simulink model "MotorTorqueControlTest_working_5_8_2022_ADC_FILT_Mo"  (R2024b)
settings: Solver=FixedStepAuto  StartTime=0.0  StopTime=inf  FixedStep=0.001  RelTol=1e-3  EnableMultiTasking=on
undefined symbols (not defined in the file): mu_X, mu_y, sigma_X, sigma_y
libraries: slrealtimeethercatlib x35, slrealtimeiplib x6, slrealtimeutilitieslib x5, simulink_extras x5, slrealtimeloglib x3, slpidlib x1, simulink x1
(part 2 of 4)

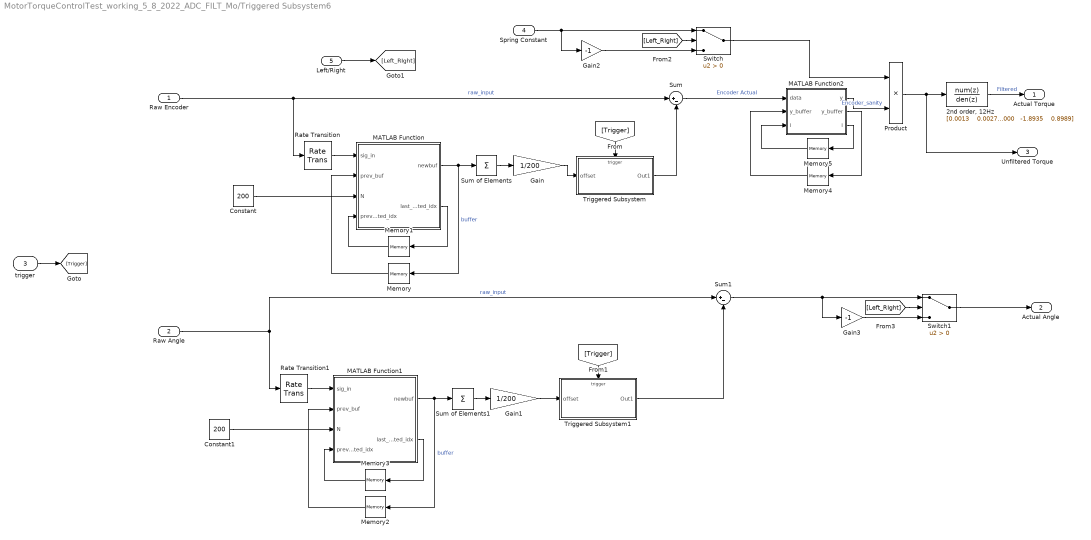
== system MotorTorqueControlTest_working_5_8_2022_ADC_FILT_Mo/Triggered Subsystem6 ==
  Raw Encoder : Inport
  Raw Angle : Inport  Port=2
  trigger : Inport  Port=3
  Spring Constant : Inport  Port=4
  Left/Right : Inport  Port=5
  "2nd order, 12Hz" : DiscreteFilter  Numerator="[0.0013    0.0027    0.0013]"  Denominator="[1.0000   -1.8935    0.8989]"
  Constant : Constant  Value=200
  Constant1 : Constant  Value=200
  Gain : Gain  Gain=1/200
  Gain1 : Gain  Gain=1/200
  Gain2 : Gain  Gain=-1
  Gain3 : Gain  Gain=-1
  MATLAB Function : MATLAB Function  TreatAsAtomicUnit=on  SystemSampleTime=1/200
  MATLAB Function1 : MATLAB Function  TreatAsAtomicUnit=on  SystemSampleTime=1/200
  MATLAB Function2 : MATLAB Function  TreatAsAtomicUnit=on
  Memory : Memory  InitialCondition=zeros(200,1)
  Memory1 : Memory
  Memory2 : Memory  InitialCondition=zeros(200,1)
  Memory3 : Memory
  Memory4 : Memory  InitialCondition=zeros(1,5)
  Memory5 : Memory
  Product : Product
  Rate Transition : RateTransition  OutPortSampleTime=1/200
  Rate Transition1 : RateTransition  OutPortSampleTime=1/200
  Sum : Sum  Inputs=|+-
  Sum of Elements : Sum  Inputs=+
  Sum of Elements1 : Sum  Inputs=+
  Sum1 : Sum  Inputs=|+-
  Switch : Switch  Criteria=u2 > Threshold  SaturateOnIntegerOverflow=off  InputSameDT=off
  Switch1 : Switch  Criteria=u2 > Threshold  SaturateOnIntegerOverflow=off  InputSameDT=off
  Triggered Subsystem : Subsystem  TreatAsAtomicUnit=on
  Triggered Subsystem1 : Subsystem  TreatAsAtomicUnit=on
  Actual Torque : Outport
  Actual Angle : Outport  Port=2
  Unfiltered Torque : Outport  Port=3
  wires:
  Rate Transition/1 -> MATLAB Function/1(sig_in)
  Memory1/1 -> MATLAB Function/4(prev_updated_idx)
  MATLAB Function/2(last_updated_idx) -> Memory1/1
  Memory/1 -> MATLAB Function/2(prev_buf)
  Constant/1 -> MATLAB Function/3(N)
  Sum of Elements/1 -> Gain/1
  Triggered Subsystem/1(Out1) -> Sum/2
  Gain/1 -> Triggered Subsystem/1(offset)
  MATLAB Function/1(newbuf) -> Memory/1, Sum of Elements/1  "buffer"
  Raw Encoder/1 -> Sum/1, Rate Transition/1  "raw_input"
  MATLAB Function1/2(last_updated_idx) -> Memory3/1
  [Trigger] -> Triggered Subsystem1/Trigger
  Memory2/1 -> MATLAB Function1/2(prev_buf)
  Gain1/1 -> Triggered Subsystem1/1(offset)
  Sum of Elements1/1 -> Gain1/1
  MATLAB Function1/1(newbuf) -> Memory2/1, Sum of Elements1/1  "buffer"
  Constant1/1 -> MATLAB Function1/3(N)
  Rate Transition1/1 -> MATLAB Function1/1(sig_in)
  Raw Angle/1 -> Sum1/1, Rate Transition1/1  "raw_input"
  Memory3/1 -> MATLAB Function1/4(prev_updated_idx)
  trigger/1 -> [Trigger]
  [Trigger] -> Triggered Subsystem/Trigger
  Triggered Subsystem1/1(Out1) -> Sum1/2
  Sum1/1 -> Gain3/1, Switch1/1
  Sum/1 -> MATLAB Function2/1(data)  "Encoder Actual"
  Product/1 -> Unfiltered Torque/1, "2nd order, 12Hz"/1
  Spring Constant/1 -> Gain2/1, Switch/1
  Memory4/1 -> MATLAB Function2/2("y_buffer ")
  "2nd order, 12Hz"/1 -> Actual Torque/1  "Filtered"
  Left/Right/1 -> [Left_RIght]
  Gain2/1 -> Switch/3
  Switch/1 -> Product/1
  Gain3/1 -> Switch1/3
  Switch1/1 -> Actual Angle/1
  [Left_RIght] -> Switch/2
  [Left_RIght] -> Switch1/2
  MATLAB Function2/2(y_buffer) -> Memory4/1
  MATLAB Function2/1(y) -> Product/2  "Encoder_sanity"
  MATLAB Function2/3(i) -> Memory5/1
  Memory5/1 -> MATLAB Function2/3("i ")

== system MotorTorqueControlTest_working_5_8_2022_ADC_FILT_Mo/RL-AAN/Triggered Subsystem ==
  note: Note: Add input/output of Critic Loss, Actor Loss, Uc, Eta, V_tderr
  In1 : Inport
  Trigger : TriggerPort  VariantControl=(inherit)
  Byte Packing : slrealtimeutilitieslib/Byte Packing  MaskPackedDataType=uint8  MaskUnpackedDataTypes={'double'}  MaskAlignment=1
  UDP Send : slrealtimeiplib/UDP Send  useHostTargetConn=off  toAddress='192.168.7.15'  toPort=5555  sampleTime=-1  enableMessage=off
  bytes : Constant  Value=8
  wires:
  Byte Packing/1 -> UDP Send/1
  bytes/1 -> UDP Send/2
  In1/1 -> Byte Packing/1

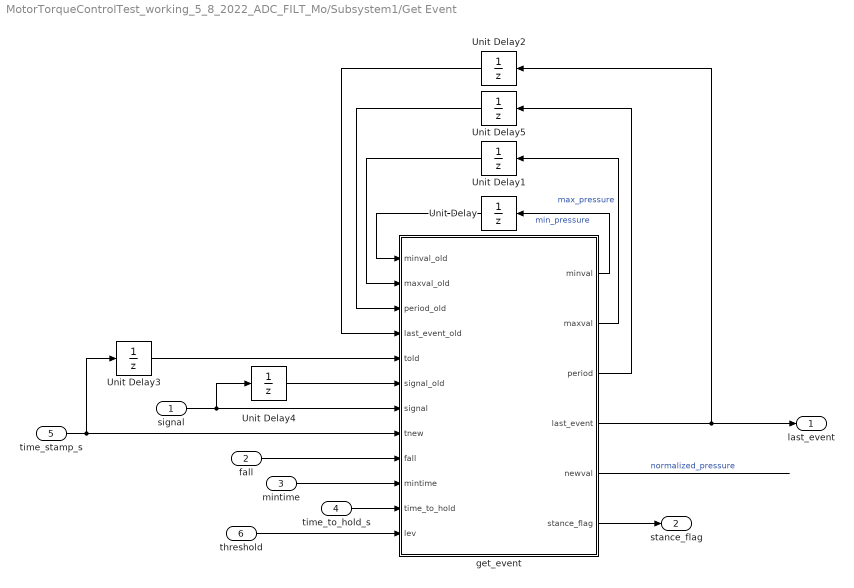
== system MotorTorqueControlTest_working_5_8_2022_ADC_FILT_Mo/Subsystem1/Get Event ==
  signal : Inport
  fall : Inport  Port=2
  mintime : Inport  Port=3
  time_to_hold_s : Inport  Port=4
  time_stamp_s : Inport  Port=5
  threshold : Inport  Port=6
  Unit Delay : UnitDelay  InitialCondition=50  SampleTime=-1
  Unit Delay1 : UnitDelay  InitialCondition=400  SampleTime=-1
  Unit Delay{2..5} (4 alike) : UnitDelay  SampleTime=-1
  get_event : MATLAB Function  TreatAsAtomicUnit=on
  last_event : Outport
  stance_flag : Outport  Port=2
  wires:
  get_event/6(stance_flag) -> stance_flag/1
  get_event/5(newval) -> ?  "normalized_pressure"
  time_stamp_s/1 -> Unit Delay3/1, get_event/8(tnew)
  Unit Delay5/1 -> get_event/3(period_old)
  signal/1 -> Unit Delay4/1, get_event/7(signal)
  get_event/3(period) -> Unit Delay5/1
  threshold/1 -> get_event/12(lev)
  Unit Delay4/1 -> get_event/6(signal_old)
  Unit Delay3/1 -> get_event/5(told)
  fall/1 -> get_event/9(fall)
  mintime/1 -> get_event/10(mintime)
  time_to_hold_s/1 -> get_event/11(time_to_hold)
  Unit Delay2/1 -> get_event/4(last_event_old)
  Unit Delay1/1 -> get_event/2(maxval_old)
  Unit Delay/1 -> get_event/1(minval_old)
  get_event/4(last_event) -> Unit Delay2/1, last_event/1
  get_event/2(maxval) -> Unit Delay1/1  "max_pressure"
  get_event/1(minval) -> Unit Delay/1  "min_pressure"

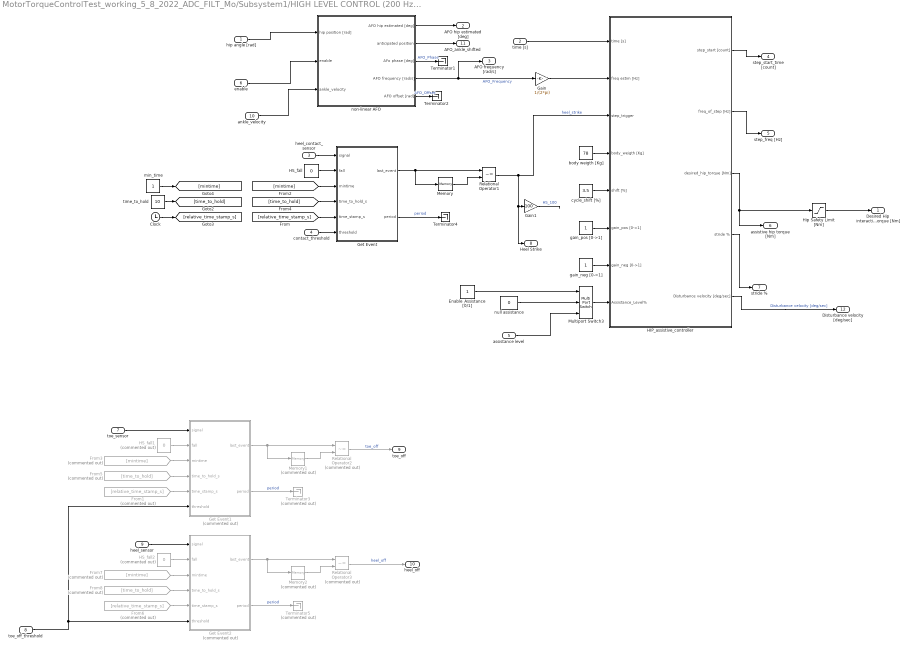
== system MotorTorqueControlTest_working_5_8_2022_ADC_FILT_Mo/Subsystem1/HIGH LEVEL CONTROL (200 Hz)1 ==
  hip angle [rad] : Inport
  time [s] : Inport  Port=2
  heel_contact_sensor : Inport  Port=3
  contact_threshold : Inport  Port=4
  assistance level : Inport  Port=5
  enable : Inport  Port=6
  toe_sensor : Inport  Port=7
  toe_off_threshold : Inport  Port=8
  heel_sensor : Inport  Port=9
  ankle_velocity : Inport  Port=10
  Clock : Clock
  Enable_Assistance [0/1] : Constant  OutMin=[0]  OutMax=[1]  SampleTime=0.01
  From1 : From  Commented=on  GotoTag=relative_time_stamp_s
      settings: CloseFcn=tagdialog Close
  From3 : From  Commented=on  GotoTag=mintime
      settings: CloseFcn=tagdialog Close
  From5 : From  Commented=on  GotoTag=time_to_hold
      settings: CloseFcn=tagdialog Close
  From6 : From  Commented=on  GotoTag=relative_time_stamp_s
      settings: CloseFcn=tagdialog Close
  From7 : From  Commented=on  GotoTag=mintime
      settings: CloseFcn=tagdialog Close
  From8 : From  Commented=on  GotoTag=time_to_hold
      settings: CloseFcn=tagdialog Close
  Gain : Gain  Gain=1/(2*pi)
  Gain1 : Gain  Gain=100
  Get Event : Subsystem  TreatAsAtomicUnit=on  SystemSampleTime=1/200
  Get Event1 : Subsystem  Commented=on  TreatAsAtomicUnit=on  SystemSampleTime=1/200
  Get Event2 : Subsystem  Commented=on  TreatAsAtomicUnit=on  SystemSampleTime=1/200
  HIP_assistive_controller : Subsystem
  HS_fall : Constant  Value=0
  HS_fall1 : Constant  Commented=on  Value=0
  HS_fall2 : Constant  Commented=on  Value=0
  Hip Safety Limit [Nm] : Saturate  UpperLimit=50  LowerLimit=-50  SampleTime=0.01
  Memory : Memory
  Memory1 : Memory  Commented=on
  Memory2 : Memory  Commented=on
  Multiport Switch3 : MultiPortSwitch  DataPortOrder=Zero-based contiguous  Inputs=2  zeroidx=on  SampleTime=0.01  SaturateOnIntegerOverflow=off  InputSameDT=off
  Relational Operator1 : RelationalOperator  Operator=~=  OutDataTypeStr=boolean  RndMeth=Simplest  InputSameDT=off
  Relational Operator2 : RelationalOperator  Commented=on  Operator=~=  OutDataTypeStr=boolean  RndMeth=Simplest  InputSameDT=off
  Relational Operator3 : RelationalOperator  Commented=on  Operator=~=  OutDataTypeStr=boolean  RndMeth=Simplest  InputSameDT=off
  Terminator1 : Terminator
  Terminator2 : Terminator
  Terminator3 : Terminator  Commented=on
  Terminator4 : Terminator
  Terminator5 : Terminator  Commented=on
  body weigth [Kg] : Constant  Value=78  OutMin=[0]  OutMax=[100]  SampleTime=0.01
  cycle_shift [%] : Constant  Value=3.5  SampleTime=0.01
  gain_neg [0->1] : Constant  OutMin=[0]  OutMax=[1]  SampleTime=0.01
  gain_pos [0->1] : Constant  OutMin=[0]  OutMax=[1]  SampleTime=0.01
  min_time : Constant
  non-linear AFO : Subsystem
  null assistance : Constant  Value=0  OutMin=[0]  OutMax=[1]  SampleTime=0.01
  time_to_hold : Constant  Value=10
  Desired Hip interaction Torque [Nm] : Outport
  AFO hip estimated [deg] : Outport  Port=2
  AFO frequency [rad/s] : Outport  Port=3
  step_start_time [count] : Outport  Port=4
  step_freq [Hz] : Outport  Port=5
  assistive hip torque [Nm] : Outport  Port=6
  stride % : Outport  Port=7
  Heel Strike : Outport  Port=8
  toe_off : Outport  Port=9
  heel_off : Outport  Port=10
  AFO_ankle_shifted : Outport  Port=11
  Disturbance velocity [deg/sec] : Outport  Port=12
  wires:
  HIP_assistive_controller/5(Disturbance velocity [deg/sec]) -> Disturbance velocity [deg/sec]/1  "Disturbance velocity [deg/sec]"
  ankle_velocity/1 -> non-linear AFO/3(ankle_velocity)
  Get Event2/2(period) -> Terminator5/1  "period"
  From8/1 -> Get Event2/4(time_to_hold_s)
  Memory2/1 -> Relational Operator3/2
  Relational Operator3/1 -> heel_off/1  "heel_off"
  heel_sensor/1 -> Get Event2/1(signal)
  Get Event2/1(last_event) -> Relational Operator3/1, Memory2/1
  From7/1 -> Get Event2/3(mintime)
  From6/1 -> Get Event2/5(time_stamp_s)
  toe_off_threshold/1 -> Get Event1/6(threshold), Get Event2/6(threshold)
  HS_fall2/1 -> Get Event2/2(fall)
  Relational Operator2/1 -> toe_off/1  "toe_off"
  From5/1 -> Get Event1/4(time_to_hold_s)
  Memory1/1 -> Relational Operator2/2
  Get Event1/1(last_event) -> Relational Operator2/1, Memory1/1
  HS_fall1/1 -> Get Event1/2(fall)
  From1/1 -> Get Event1/5(time_stamp_s)
  toe_sensor/1 -> Get Event1/1(signal)
  Get Event1/2(period) -> Terminator3/1  "period"
  From3/1 -> Get Event1/3(mintime)
  enable/1 -> non-linear AFO/2(enable)
  Gain1/1 -> ?  "HS_100"
  hip angle [rad]/1 -> non-linear AFO/1(hip position [rad])
  heel_contact_sensor/1 -> Get Event/1(signal)
  time_to_hold/1 -> [time_to_hold]
  [relative_time_stamp_s] -> Get Event/5(time_stamp_s)
  [mintime] -> Get Event/3(mintime)
  [time_to_hold] -> Get Event/4(time_to_hold_s)
  contact_threshold/1 -> Get Event/6(threshold)
  Clock/1 -> [relative_time_stamp_s]
  min_time/1 -> [mintime]
  Get Event/2(period) -> Terminator4/1  "period"
  Get Event/1(last_event) -> Relational Operator1/1, Memory/1
  Memory/1 -> Relational Operator1/2
  Relational Operator1/1 -> HIP_assistive_controller/3(step_trigger), Gain1/1, Heel Strike/1  "heel_strike"
  HS_fall/1 -> Get Event/2(fall)
  assistance level/1 -> Multiport Switch3/3
  Multiport Switch3/1 -> HIP_assistive_controller/8(Assistance_Level%)
  gain_pos [0->1]/1 -> HIP_assistive_controller/6(gain_pos [0->1])
  non-linear AFO/5(AFO offset [rad]) -> Terminator2/1  "AFO_Offset"
  non-linear AFO/3(AFo phase [deg]) -> Terminator1/1  "AFO_Phase"
  non-linear AFO/2(anticipated position) -> AFO_ankle_shifted/1
  null assistance/1 -> Multiport Switch3/2
  Enable_Assistance [0/1]/1 -> Multiport Switch3/1
  gain_neg [0->1]/1 -> HIP_assistive_controller/7(gain_neg [0->1])
  cycle_shift [%]/1 -> HIP_assistive_controller/5(shift [%])
  body weigth [Kg]/1 -> HIP_assistive_controller/4(body_weigth [Kg])
  HIP_assistive_controller/4(stride %) -> stride %/1
  HIP_assistive_controller/3(desired_hip_torque [Nm]) -> assistive hip torque [Nm]/1, Hip Safety Limit [Nm]/1
  HIP_assistive_controller/2(freq_of_step [Hz]) -> step_freq [Hz]/1
  HIP_assistive_controller/1(step_start [count]) -> step_start_time [count]/1
  time [s]/1 -> HIP_assistive_controller/1(time [s])
  Gain/1 -> HIP_assistive_controller/2(freq estim [Hz])
  non-linear AFO/4(AFO frequency [rad/s]) -> AFO frequency [rad/s]/1, Gain/1  "AFO_Frequency"
  non-linear AFO/1(AFO hip estimated [deg]) -> AFO hip estimated [deg]/1
  Hip Safety Limit [Nm]/1 -> Desired Hip interaction Torque [Nm]/1

== system MotorTorqueControlTest_working_5_8_2022_ADC_FILT_Mo/Subsystem1/stride % calculation ==
  step_trigger : Inport
  timer : Inport  Port=2
  step_freq_estimated : Inport  Port=3
  Product1 : Product  RndMeth=Zero
  Sum : Sum  Inputs=|-+
  take step start and period : Subsystem  TreatAsAtomicUnit=on
  to% : Gain  Gain=100
  stride % : Outport
  wires:
  to%/1 -> stride %/1
  step_trigger/1 -> take step start and period/Trigger
  timer/1 -> take step start and period/1(time_counter), Sum/2
  take step start and period/1(time_count_stepon) -> Sum/1
  step_freq_estimated/1 -> Product1/2
  Sum/1 -> Product1/1
  Product1/1 -> to%/1

== system MotorTorqueControlTest_working_5_8_2022_ADC_FILT_Mo/Triggered Subsystem6/Triggered Subsystem ==
  offset : Inport
  Trigger : TriggerPort  VariantControl=(inherit)
  Out1 : Outport
  wires:
  offset/1 -> Out1/1

== system MotorTorqueControlTest_working_5_8_2022_ADC_FILT_Mo/Triggered Subsystem6/Triggered Subsystem1 ==
  offset : Inport
  Trigger : TriggerPort  VariantControl=(inherit)
  Out1 : Outport
  wires:
  offset/1 -> Out1/1

== system MotorTorqueControlTest_working_5_8_2022_ADC_FILT_Mo/Subsystem1/HIGH LEVEL CONTROL (200 Hz)1/Get Event ==
  signal : Inport
  fall : Inport  Port=2
  mintime : Inport  Port=3
  time_to_hold_s : Inport  Port=4
  time_stamp_s : Inport  Port=5
  threshold : Inport  Port=6
  Unit Delay{,2..5} (5 alike) : UnitDelay  SampleTime=-1
  Unit Delay1 : UnitDelay  InitialCondition=-1000  SampleTime=-1
  get_event : MATLAB Function  TreatAsAtomicUnit=on
  last_event : Outport
  period : Outport  Port=2
  wires:
  get_event/5(newval) -> ?  "normalized_pressure"
  time_stamp_s/1 -> Unit Delay3/1, get_event/8(tnew)
  Unit Delay5/1 -> get_event/3(period_old)
  signal/1 -> Unit Delay4/1, get_event/7(signal)
  get_event/3(period) -> Unit Delay5/1, period/1
  threshold/1 -> get_event/12(lev)
  Unit Delay4/1 -> get_event/6(signal_old)
  Unit Delay3/1 -> get_event/5(told)
  fall/1 -> get_event/9(fall)
  mintime/1 -> get_event/10(mintime)
  time_to_hold_s/1 -> get_event/11(time_to_hold)
  Unit Delay2/1 -> get_event/4(last_event_old)
  Unit Delay1/1 -> get_event/2(maxval_old)
  Unit Delay/1 -> get_event/1(minval_old)
  get_event/4(last_event) -> Unit Delay2/1, last_event/1
  get_event/2(maxval) -> Unit Delay1/1  "max_pressure"
  get_event/1(minval) -> Unit Delay/1  "min_pressure"

== system MotorTorqueControlTest_working_5_8_2022_ADC_FILT_Mo/Subsystem1/HIGH LEVEL CONTROL (200 Hz)1/Get Event1 ==
  signal : Inport
  fall : Inport  Port=2
  mintime : Inport  Port=3
  time_to_hold_s : Inport  Port=4
  time_stamp_s : Inport  Port=5
  threshold : Inport  Port=6
  Unit Delay : UnitDelay  InitialCondition=4.5  SampleTime=-1
  Unit Delay1 : UnitDelay  InitialCondition=0.5  SampleTime=-1
  Unit Delay{2..5} (4 alike) : UnitDelay  SampleTime=-1
  get_event : MATLAB Function  TreatAsAtomicUnit=on
  last_event : Outport
  period : Outport  Port=2
  wires:
  time_stamp_s/1 -> Unit Delay3/1, get_event/8(tnew)
  Unit Delay5/1 -> get_event/3(period_old)
  signal/1 -> Unit Delay4/1, get_event/7(signal)
  get_event/3(period) -> period/1, Unit Delay5/1
  threshold/1 -> get_event/12(lev)
  Unit Delay4/1 -> get_event/6(signal_old)
  Unit Delay3/1 -> get_event/5(told)
  fall/1 -> get_event/9(fall)
  mintime/1 -> get_event/10(mintime)
  time_to_hold_s/1 -> get_event/11(time_to_hold)
  Unit Delay2/1 -> get_event/4(last_event_old)
  Unit Delay1/1 -> get_event/2(maxval_old)
  Unit Delay/1 -> get_event/1(minval_old)
  get_event/4(last_event) -> last_event/1, Unit Delay2/1
  get_event/2(maxval) -> Unit Delay1/1
  get_event/1(minval) -> Unit Delay/1

== system MotorTorqueControlTest_working_5_8_2022_ADC_FILT_Mo/Subsystem1/HIGH LEVEL CONTROL (200 Hz)1/Get Event2 ==
  signal : Inport
  fall : Inport  Port=2
  mintime : Inport  Port=3
  time_to_hold_s : Inport  Port=4
  time_stamp_s : Inport  Port=5
  threshold : Inport  Port=6
  Unit Delay : UnitDelay  InitialCondition=4.5  SampleTime=-1
  Unit Delay1 : UnitDelay  InitialCondition=0.5  SampleTime=-1
  Unit Delay{2..5} (4 alike) : UnitDelay  SampleTime=-1
  get_event : MATLAB Function  TreatAsAtomicUnit=on
  last_event : Outport
  period : Outport  Port=2
  wires:
  time_stamp_s/1 -> Unit Delay3/1, get_event/8(tnew)
  Unit Delay5/1 -> get_event/3(period_old)
  signal/1 -> Unit Delay4/1, get_event/7(signal)
  get_event/3(period) -> period/1, Unit Delay5/1
  threshold/1 -> get_event/12(lev)
  Unit Delay4/1 -> get_event/6(signal_old)
  Unit Delay3/1 -> get_event/5(told)
  fall/1 -> get_event/9(fall)
  mintime/1 -> get_event/10(mintime)
  time_to_hold_s/1 -> get_event/11(time_to_hold)
  Unit Delay2/1 -> get_event/4(last_event_old)
  Unit Delay1/1 -> get_event/2(maxval_old)
  Unit Delay/1 -> get_event/1(minval_old)
  get_event/4(last_event) -> last_event/1, Unit Delay2/1
  get_event/2(maxval) -> Unit Delay1/1
  get_event/1(minval) -> Unit Delay/1

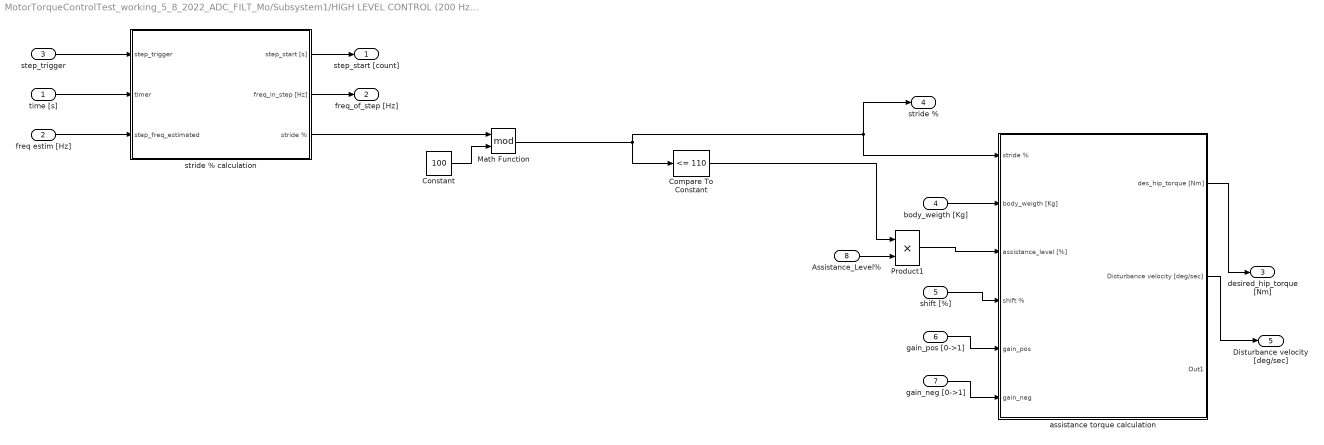
== system MotorTorqueControlTest_working_5_8_2022_ADC_FILT_Mo/Subsystem1/HIGH LEVEL CONTROL (200 Hz)1/HIP_assistive_controller ==
  time [s] : Inport
  freq estim [Hz] : Inport  Port=2
  step_trigger : Inport  Port=3
  body_weigth [Kg] : Inport  Port=4
  shift [%] : Inport  Port=5
  gain_pos [0->1] : Inport  Port=6
  gain_neg [0->1] : Inport  Port=7
  Assistance_Level% : Inport  Port=8
  Compare To Constant : simulink/Logic and Bit Operations/Compare To Constant  relop=<=  const=110  OutDataTypeStr=uint8
  Constant : Constant  Value=100
  Math Function : Math  Operator=mod
  Product1 : Product  RndMeth=Zero  SampleTime=0.01
  assistance torque calculation : Subsystem
  stride % calculation : Subsystem
  step_start [count] : Outport
  freq_of_step [Hz] : Outport  Port=2
  desired_hip_torque [Nm] : Outport  Port=3
  stride % : Outport  Port=4
  Disturbance velocity [deg/sec] : Outport  Port=5
  wires:
  assistance torque calculation/2(Disturbance velocity [deg/sec]) -> Disturbance velocity [deg/sec]/1
  Constant/1 -> Math Function/2
  stride % calculation/3(stride %) -> Math Function/1
  Assistance_Level%/1 -> Product1/2
  Product1/1 -> assistance torque calculation/3(assistance_level [%])
  gain_neg [0->1]/1 -> assistance torque calculation/6(gain_neg)
  gain_pos [0->1]/1 -> assistance torque calculation/5(gain_pos)
  shift [%]/1 -> assistance torque calculation/4(shift %)
  Compare To Constant/1 -> Product1/1
  assistance torque calculation/1(des_hip_torque [Nm]) -> desired_hip_torque [Nm]/1
  freq estim [Hz]/1 -> stride % calculation/3(step_freq_estimated)
  stride % calculation/2(freq_in_step [Hz]) -> freq_of_step [Hz]/1
  time [s]/1 -> stride % calculation/2(timer)
  stride % calculation/1(step_start [s]) -> step_start [count]/1
  step_trigger/1 -> stride % calculation/1(step_trigger)
  Math Function/1 -> Compare To Constant/1, stride %/1, assistance torque calculation/1(stride %)
  body_weigth [Kg]/1 -> assistance torque calculation/2(body_weigth [Kg])

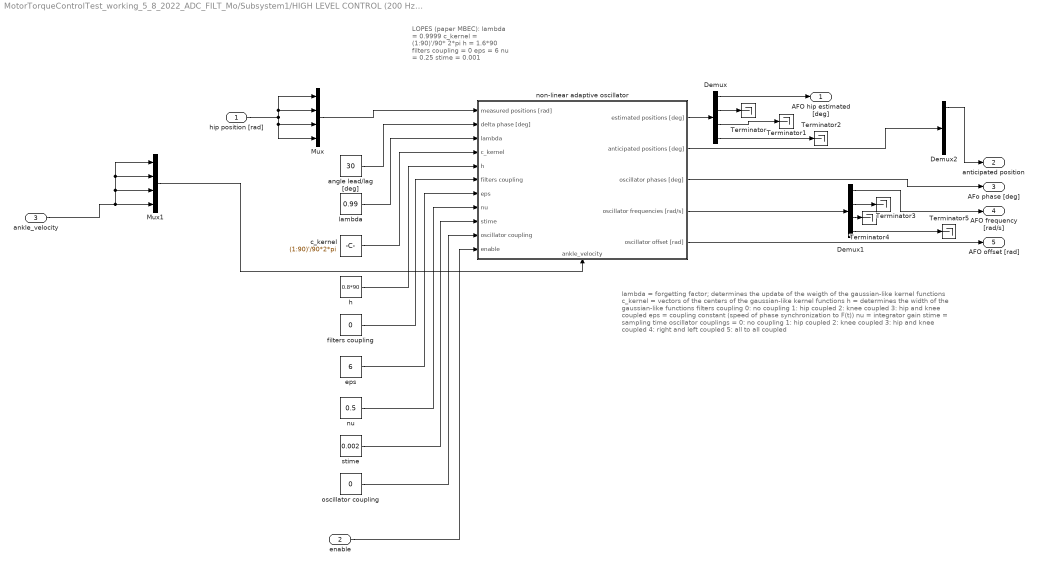
== system MotorTorqueControlTest_working_5_8_2022_ADC_FILT_Mo/Subsystem1/HIGH LEVEL CONTROL (200 Hz)1/non-linear AFO ==
  note: lambda = forgetting factor; determines the update of the weigth of the gaussian-like kernel functions
      | c_kernel = vectors of the centers of the gaussian-like kernel functions
      | h = determines the width of the gaussian-like functions
      | filters coupling
      | 0: no coupling
      | 1: hip coupled
      | 2: knee coupled
      | 3: hip and knee coupled
      | eps = coupling constant (speed of phase synchronization to F(t))
      | nu = integrator gain
      | stime = sampling time
      | oscillator couplings =
      | 0: no coupling
      | 1: hip coupled
      | 2: knee coupled
      | 3: hip and knee coupled
      | 4: right and left coupled
      | 5: all to all coupled
  note: LOPES (paper MBEC):
      | lambda = 0.9999
      | c_kernel = (1:90)'/90* 2*pi
      | h = 1.6*90
      | filters coupling = 0
      | eps = 6
      | nu = 0.25
      | stime = 0.001
  hip position [rad] : Inport
  enable : Inport  Port=2
  ankle_velocity : Inport  Port=3
  Demux : Demux
  Demux1 : Demux
  Demux2 : Demux
  Mux : Mux
  Mux1 : Mux
  Terminator{,1..5} (6 alike) : Terminator
  angle lead/lag [deg] : Constant  Value=30  SampleTime=0.01
  c_kernel : Constant  Value=(1:90)'/90*2*pi  SampleTime=0.01
  eps : Constant  Value=6  SampleTime=0.01
  filters coupling : Constant  Value=0  SampleTime=0.01
  h : Constant  Value=0.8*90  SampleTime=0.01
  lambda : Constant  Value=0.99  SampleTime=0.01
  non-linear adaptive oscillator : Subsystem
      settings: PortSchema="{\"entries\":[{\"content\":{\"sides\":[{\"content\":{\"connectorIds\":[\"In1\",\"In2\",\"In3\",\"In4\",\"In5\",\"In6\",\"In7\",\"In8\",\"In9\",\"In10\",\"In11\"]},\"type\":\"ConnectorPlacement.EquallySpacedRectSide\",\"uuid\":\"ab3a5fe0-9bb0-482e-b44f-9f3ccb1731cf\"},{\"content\":{\"connectorIds\":[\"Out1\",\"Out2\",\"Out3\",\"Out4\",\"Out5\"],\"side\":\"RIGHT\"},\"type\":\"ConnectorPlacement.EquallySpacedRectSide\",\"uuid\":\"96980b87-f654-464e-8cdf-49c302ee1131\"},{\"content\":{\"connectorIds\":[],\"side\":\"TOP\"},\"type\":\"ConnectorPlacement.EquallySpacedRectSide\",\"uuid\":\"71bd0918-5e69-4492-a5e8-d47966924c89\"},{\"content\":{\"connectorIds\":[\"In12\"],\"side\":\"BOTTOM\"},\"type\":\"ConnectorPlacement.EquallySpacedRectSide\",\"uuid\":\"e65d897a-cb77-4120-a9be-e238fcdd4933\"}]},\"type\":\"ConnectorPlacement.EquallySpacedConnector\",\"uuid\":\"727f1d0f-0b0c-4f59-bcfa-1816f6ded572\"}],\"packageUris\":[\"http://schema.mathworks.com/mf0/Connector/R2020b\"],\"version\":\"1.0\"}"
  nu : Constant  Value=0.5  SampleTime=0.01
  oscillator coupling : Constant  Value=0  SampleTime=0.01
  stime : Constant  Value=0.002  SampleTime=0.01
  AFO hip estimated [deg] : Outport
  anticipated position : Outport  Port=2
  AFo phase [deg] : Outport  Port=3
  AFO frequency [rad/s] : Outport  Port=4
  AFO offset [rad] : Outport  Port=5
  wires:
  Mux1/1 -> non-linear adaptive oscillator/12(ankle_velocity)
  ankle_velocity/1 -> Mux1/4, Mux1/2, Mux1/1, Mux1/3
  Demux2/1 -> anticipated position/1
  enable/1 -> non-linear adaptive oscillator/11(enable)
  Demux1/4 -> Terminator5/1
  Demux1/3 -> Terminator4/1
  Demux1/2 -> Terminator3/1
  Demux/4 -> Terminator2/1
  Demux/3 -> Terminator1/1
  Demux/2 -> Terminator/1
  Demux1/1 -> AFO frequency [rad/s]/1
  non-linear adaptive oscillator/4(oscillator frequencies [rad/s]) -> Demux1/1
  non-linear adaptive oscillator/5(oscillator offset [rad]) -> AFO offset [rad]/1
  non-linear adaptive oscillator/3(oscillator phases [deg]) -> AFo phase [deg]/1
  non-linear adaptive oscillator/2(anticipated positions [deg]) -> Demux2/1
  hip position [rad]/1 -> Mux/3, Mux/4, Mux/2, Mux/1
  Demux/1 -> AFO hip estimated [deg]/1
  non-linear adaptive oscillator/1(estimated positions [deg]) -> Demux/1
  Mux/1 -> non-linear adaptive oscillator/1(measured positions [rad])
  oscillator coupling/1 -> non-linear adaptive oscillator/10(oscillator coupling)
  nu/1 -> non-linear adaptive oscillator/8(nu)
  stime/1 -> non-linear adaptive oscillator/9(stime)
  eps/1 -> non-linear adaptive oscillator/7(eps)
  filters coupling/1 -> non-linear adaptive oscillator/6(filters coupling)
  h/1 -> non-linear adaptive oscillator/5(h)
  c_kernel/1 -> non-linear adaptive oscillator/4(c_kernel)
  lambda/1 -> non-linear adaptive oscillator/3(lambda)
  angle lead/lag [deg]/1 -> non-linear adaptive oscillator/2(delta phase [deg])

== system MotorTorqueControlTest_working_5_8_2022_ADC_FILT_Mo/Subsystem1/stride % calculation/take step start and period ==
  time_counter : Inport
  Trigger : TriggerPort  VariantControl=(inherit)
  time_count_stepon : Outport
  wires:
  time_counter/1 -> time_count_stepon/1

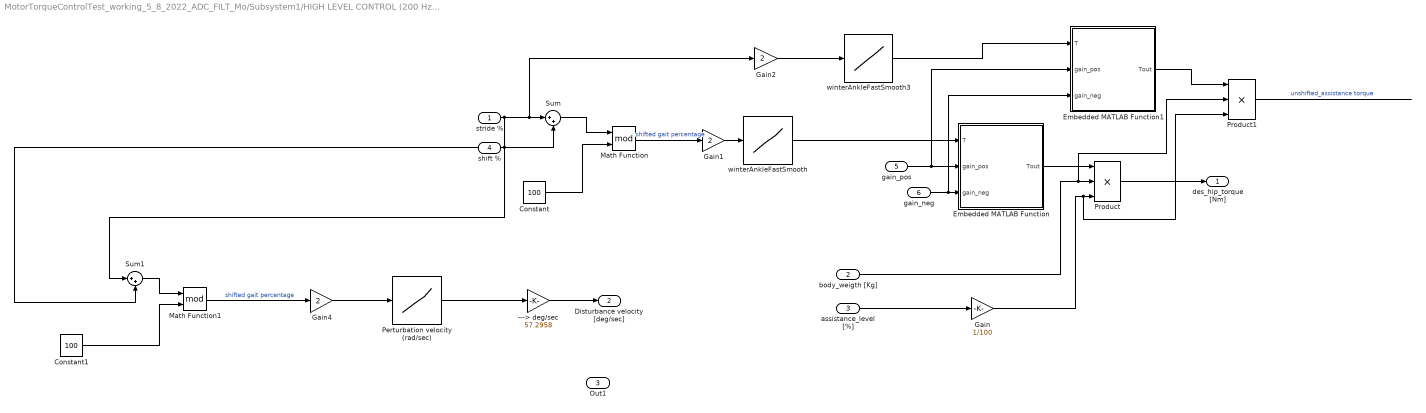
== system MotorTorqueControlTest_working_5_8_2022_ADC_FILT_Mo/Subsystem1/HIGH LEVEL CONTROL (200 Hz)1/HIP_assistive_controller/assistance torque calculation ==
  stride % : Inport
  body_weigth [Kg] : Inport  Port=2
  assistance_level [%] : Inport  Port=3
  shift % : Inport  Port=4
  gain_pos : Inport  Port=5
  gain_neg : Inport  Port=6
  ---> deg/sec : Gain  Gain=57.2958
  Constant : Constant  Value=100
  Constant1 : Constant  Value=100
  Embedded MATLAB Function : MATLAB Function  TreatAsAtomicUnit=on
  Embedded MATLAB Function1 : MATLAB Function  TreatAsAtomicUnit=on
  Gain : Gain  Gain=1/100  SampleTime=0.01
  Gain1 : Gain  Gain=2
  Gain2 : Gain  Gain=2
  Gain4 : Gain  Gain=2
  Math Function : Math  Operator=mod
  Math Function1 : Math  Operator=mod
  Perturbation velocity (rad/sec) : Lookup  InputValues=[0:199]  Table="[-4.93270593173997e-253\t4.04481886402677e-252\t-2.92815289519947e-249\t2.11997865130555e-246\t-1.53486161539233e-243\t1.11123768956540e-240\t-8.04534552383726e-238\t5.82481904688132e-235\t-4.21716094459655e-232\t3.05321869906885e-229\t-2.21052612096491e-226\t1.60041785835989e-223\t-1.15870031892643e-220\t8.38897430484885e-218\t-6.07360580970738e-215\t4.39728221725384e-212\t-3.18362625168597e-209\t2.30494100893842e-206\t-1.66877410684517e-203\t1.20819014841489e-200\t-8.74727998678275e-198\t6.33301862852906e-195\t-4.58509673977517e-192\t3.31960370657860e-189\t-2.40338849846610e-186\t1.74004995328580e-183\t-1.25979376279042e-180\t9.12088944210309e-178\t-6.60351135814501e-175\t4.78093310240728e-172\t-3.46138896263170e-169\t2.50604082801225e-166\t-1.81437009809191e-163\t1.31360144497771e-160\t-9.51045631793764e-158\t6.88555723817240e-155\t-4.98513392998050e-152\t3.60923007974864e-149\t-2.61307759260409e-146\t1.89186456781528e-143\t-1.36970733402067e-140\t9.91666217966397e-138\t-7.17964972100335e-135\t5.19805648134426e-132\t-3.76338571284352e-129\t2.72468605804223e-126\t-1.97266894263686e-123\t1.42820958978303e-120\t-1.03402177033392e-117\t7.48630333512205e-115\t-5.42007327441066e-112\t3.92412556436998e-109\t-2.84106148853059e-106\t2.05692459357058e-103\t-1.48921056468361e-100\t1.07818639190634e-97\t-7.80605458529627e-95\t5.65157273789058e-92\t-4.09173085617816e-89\t2.96240748830027e-86\t-2.14477892979854e-83\t1.55281698276666e-80\t-1.12423735074413e-77\t8.13946289121766e-75\t-5.89295989086808e-72\t4.26649482152560e-69\t-3.08893635782464e-66\t2.23638565657022e-63\t-1.61914012642048e-60\t1.17225521514277e-57\t-8.48711156623239e-55\t6.14465705140010e-52\t-4.44872321810211e-49\t3.22086946524887e-46\t-2.33190504411696e-43\t1.68829603107122e-40\t-1.22232399459052e-37\t8.84960883787503e-35\t-6.40710457538158e-32\t4.63873486296742e-29\t-3.35843763368384e-26\t2.43150420805224e-23\t-1.76040568819219e-20\t1.27453128674693e-17\t-9.22758891199092e-15\t6.68076162696856e-12\t-4.83686219033632e-09\t3.50188154504187e-06\t-0.00626761298606990\t-0.0765669636741737\t-0.159007648472814\t-0.255697732492699\t-0.366569255690371\t-0.490682383459649\t-0.627060602245939\t-0.775477718863351\t-0.936729568178100\t-1.11230265194788\t-1.30336585588083\t-1.50962253596126\t-1.72869176641761\t-1.95637366717679\t-2.18811628055900\t-2.42034717099672\t-2.65047734470819\t-2.87635971143045\t-3.09600015053043\t-3.30729754329227\t-3.50752844204451\t-3.69318852845936\t-3.86078591589950\t-4.00765115546246\t-4.13182288263306\t-4.23158106680777\t-4.30521091005464\t-4.35074237213917\t-4.36540997346769\t-4.34542368201912\t-4.28664128375527\t-4.18519646810363\t-4.03727504299778\t-3.83904583007861\t-3.58777079098347\t-3.28337600797458\t-2.93062745352010\t-1.28036789819353\t0.00132410560966730\t-1.82887864053534e-06\t2.52608028950714e-09\t-3.48906782965580e-12\t4.81916365465694e-15\t-6.65631608906347e-18\t9.19382429245723e-21\t-1.26986765636748e-23\t1.75396419747845e-26\t-2.42260710445788e-29\t3.34614879311990e-32\t-4.62176129389610e-35\t6.38366037447886e-38\t-8.81722728314056e-41\t1.21785139562475e-43\t-1.68211839640513e-46\t2.32337238327194e-49\t-3.20908399960916e-52\t4.43244491958885e-55\t-6.12217317078076e-58\t8.45605642325827e-61\t-1.16796582257095e-63\t1.61321553974235e-66\t-2.22820251018784e-69\t3.07763364788833e-72\t-4.25088331393000e-75\t5.87139699393623e-78\t-8.10967982758677e-81\t1.12012366007425e-83\t-1.54713507873650e-86\t2.13693098108324e-89\t-2.95156775945036e-92\t4.07675882644125e-95\t-5.63089309935420e-98\t7.77749149415344e-101\t-1.07424120604507e-103\t1.48376140254605e-106\t-2.04939811217073e-109\t2.83066577615762e-112\t-3.90976681822861e-115\t5.40024071428065e-118\t-7.45891024400900e-121\t1.03023818699522e-123\t-1.42298363597511e-126\t1.96545076062331e-129\t-2.71471617436249e-132\t3.74961512900386e-135\t-5.17903630163337e-138\t7.15337870443307e-141\t-9.88037617594962e-144\t1.36469544549312e-146\t-1.88494205664256e-149\t2.60351609484272e-152\t-3.59602356593311e-155\t4.96689285399923e-158\t-6.86036233377885e-161\t9.47565665984445e-164\t-1.30879485319833e-166\t1.80773114650458e-169\t-2.49687098788397e-172\t3.44872341342956e-175\t-4.76343921654497e-178\t6.57934848626995e-181\t-9.08751524600982e-184\t1.25518405840322e-186\t-1.73368294612913e-189\t2.39459427290897e-192\t-3.30745696302266e-195\t4.56831943766322e-198\t-6.30984551510508e-201\t8.71527286298032e-204\t-1.20376926652754e-206\t1.66266790505841e-209\t-2.29673474975219e-212]"  SaturateOnIntegerOverflow=off
  Product : Product  Inputs=3  RndMeth=Zero
  Product1 : Product  Inputs=3  RndMeth=Zero
  Sum : Sum  Inputs=|++
  Sum1 : Sum  Inputs=|++
  winterAnkleFastSmooth : Lookup  InputValues=[0:200]  Table="[0\t0\t0\t0\t0\t0\t0\t0\t0\t0\t0\t0\t0\t0\t0\t0\t0\t0\t0.0123629052736435\t0.0412585090601981\t0.0720000000000000\t0.104333911147289\t0.137883548612989\t0.172241411772194\t0.207000000000000\t0.241722256560577\t0.275852900274400\t0.308807093851024\t0.340000000000000\t0.368933312610405\t0.395454850289409\t0.419498962823709\t0.441000000000000\t0.459966367997805\t0.476702698567963\t0.491587679854139\t0.505000000000000\t0.517248090398375\t0.528359355438741\t0.538290942759736\t0.547000000000000\t0.554463145408695\t0.560734879677075\t0.565889174106917\t0.570000000000000\t0.573149327966846\t0.575451125852960\t0.577027360812594\t0.578000000000000\t0.578502042723923\t0.578710616911085\t0.578813882642705\t0.579000000000000\t0.579451876137464\t0.580331406502699\t0.581795233616584\t0.584000000000000\t0.587112327726223\t0.591338757078120\t0.596895807890957\t0.604000000000000\t0.612880062957646\t0.623813565184823\t0.637090284819588\t0.653000000000000\t0.671711170443192\t0.692906982182590\t0.716149302830693\t0.741000000000000\t0.767228380269585\t0.795433506084817\t0.826421878857641\t0.861000000000000\t0.899672183478468\t0.941733993478140\t0.986178806738742\t1.03200000000000\t1.07844226081654\t1.12575552000262\t1.17444101918739\t1.22500000000000\t1.27765252325536\t1.33149392651137\t1.38533836651170\t1.43800000000000\t1.48843202116203\t1.53614377395190\t1.58078363976582\t1.62200000000000\t1.65933814209653\t1.69193097768103\t1.71880832442502\t1.73900000000000\t1.75165291045186\t1.75638231532399\t1.75292056253412\t1.74100000000000\t1.72026896609601\t1.69003976102303\t1.64954067543852\t1.59800000000000\t1.53500560016408\t1.46158364058391\t1.37911986071179\t1.28900000000000\t1.19256800824768\t1.09100067664133\t0.985433006714323\t0.877000000000000\t0.767175491845209\t0.658788652850752\t0.555007487430919\t0.459000000000000\t0.373308149371486\t0.297969711955659\t0.232396418562003\t0.176000000000000\t0.128170035668849\t0.0882074993266129\t0.0553912133210702\t0.0290000000000000\t0.00830858295311821\t-0.00742470926211037\t-0.0189456468462838\t-0.0270000000000000\t-0.0322793674813219\t-0.0352586622781714\t-0.0363586259359352\t-0.0360000000000000\t-0.0345973630278306\t-0.0325406416252041\t-0.0302135994099755\t-0.0280000000000000\t-0.0261905554073556\t-0.0247037712210123\t-0.0233651014241628\t-0.0220000000000000\t-0.0204841653427468\t-0.0188942734907467\t-0.0173572448933732\t-0.0160000000000000\t-0.0149196582216572\t-0.0140941348160010\t-0.0134715440023443\t-0.0130000000000000\t-0.0126340767706245\t-0.0123541872452493\t-0.0121472040972494\t-0.0120000000000000\t-0.0119034096958447\t-0.0118641162030018\t-0.0118927646086579\t-0.0120000000000000\t-0.0121897844459966\t-0.0124393479427436\t-0.0127192374681188\t-0.0130000000000000\t-0.0132593275201690\t-0.0135034920260239\t-0.0137459105188668\t-0.0140000000000000\t-0.0142729054733275\t-0.0145466839531609\t-0.0147971204564139\t-0.0150000000000000\t-0.0151334255865212\t-0.0151847721613325\t-0.0151437326554777\t-0.0150000000000000\t-0.0147402671805879\t-0.0143392274015089\t-0.0137685739216755\t-0.0130000000000000\t-0.0120148806911273\t-0.0108333182326318\t-0.00948509665782044\t-0.00800000000000000\t-0.00640333505490292\t-0.00470249966796380\t-0.00290041444704278\t-0.00100000000000000\t0.000987595910738992\t0.00301831690448703\t0.00503987944599156\t0.00700000000000000\t0.00884357641194696\t0.0105042320500157\t0.0119127716630766\t0.0130000000000000\t0.0137162234414732\t0.0140897548954503\t0.0141684089017022\t0.0140000000000000\t0.0136196548221603\t0.0130117483681832\t0.0121479677301145\t0.0110000000000000\t0.00953953226988547\t0.00773825163181676\t0.00556784517783966\t0.00300000000000000]"  SaturateOnIntegerOverflow=off
  winterAnkleFastSmooth3 : Lookup  InputValues=[0:200]  Table=|  SaturateOnIntegerOverflow=off
      | [-0.00700000000000000
      | -0.00198044104598932
      | -0.00904907548113065
      | -0.0250931721757067
      | -0.0470000000000000
      | -0.0716568278242934
      | -0.0959509245188694
      | -0.116769558954011
      | -0.131000000000000
      | -0.136360997656837
      | -0.133897226443392
      | -0.125484842008251
      | -0.113000000000000
      | -0.0979929315483575
      | -0.0807101697075629
      | -0.0610723230129869
      | -0.0390000000000000
      | -0.0144641511497329
      | 0.0123629052736435
      | 0.0412585090601981
      | 0.0720000000000000
      | 0.104333911147289
      | 0.137883548612989
      | 0.172241411772194
      | 0.207000000000000
      | 0.241722256560577
      | 0.275852900274400
      | 0.308807093851024
      | 0.340000000000000
      | 0.368933312610405
      | 0.395454850289409
      | 0.419498962823709
      | 0.441000000000000
      | 0.459966367997805
      | 0.476702698567963
      | 0.491587679854139
      | 0.505000000000000
      | 0.517248090398375
      | 0.528359355438741
      | 0.538290942759736
      | 0.547000000000000
      | 0.554463145408695
      | 0.560734879677075
      | 0.565889174106917
      | 0.570000000000000
      | 0.573149327966846
      | 0.575451125852960
      | 0.577027360812594
      | 0.578000000000000
      | 0.578502042723923
      | 0.578710616911085
      | 0.578813882642705
      | 0.579000000000000
      | 0.579451876137464
      | 0.580331406502699
      | 0.581795233616584
      | 0.584000000000000
      | 0.587112327726223
      | 0.591338757078120
      | 0.596895807890957
      | 0.604000000000000
      | 0.612880062957646
      | 0.623813565184823
      | 0.637090284819588
      | 0.653000000000000
      | 0.671711170443192
      | 0.692906982182590
      | 0.716149302830693
      | 0.741000000000000
      | 0.767228380269585
      | 0.795433506084817
      | 0.826421878857641
      | 0.861000000000000
      | 0.899672183478468
      | 0.941733993478140
      | 0.986178806738742
      | 1.03200000000000
      | 1.07844226081654
      | 1.12575552000262
      | 1.17444101918739
      | 1.22500000000000
      | 1.27765252325536
      | 1.33149392651137
      | 1.38533836651170
      | 1.43800000000000
      | 1.48843202116203
      | 1.53614377395190
      | 1.58078363976582
      | 1.62200000000000
      | 1.65933814209653
      | 1.69193097768103
      | 1.71880832442502
      | 1.73900000000000
      | 1.75165291045186
      | 1.75638231532399
      | 1.75292056253412
      | 1.74100000000000
      | 1.72026896609601
      | 1.69003976102303
      | 1.64954067543852
      | 1.59800000000000
      | 1.53500560016408
      | 1.46158364058391
      | 1.37911986071179
      | 1.28900000000000
      | 1.19256800824768
      | 1.09100067664133
      | 0.985433006714323
      | 0.877000000000000
      | 0.767175491845209
      | 0.658788652850752
      | 0.555007487430919
      | 0.459000000000000
      | 0.373308149371486
      | 0.297969711955659
      | 0.232396418562003
      | 0.176000000000000
      | 0.128170035668849
      | 0.0882074993266129
      | 0.0553912133210702
      | 0.0290000000000000
      | 0.00830858295311821
      | -0.00742470926211037
      | -0.0189456468462838
      | -0.0270000000000000
      | -0.0322793674813219
      | -0.0352586622781714
      | -0.0363586259359352
      | -0.0360000000000000
      | -0.0345973630278306
      | -0.0325406416252041
      | -0.0302135994099755
      | -0.0280000000000000
      | -0.0261905554073556
      | -0.0247037712210123
      | -0.0233651014241628
      | -0.0220000000000000
      | -0.0204841653427468
      | -0.0188942734907467
      | -0.0173572448933732
      | -0.0160000000000000
      | -0.0149196582216572
      | -0.0140941348160010
      | -0.0134715440023443
      | -0.0130000000000000
      | -0.0126340767706245
      | -0.0123541872452493
      | -0.0121472040972494
      | -0.0120000000000000
      | -0.0119034096958447
      | -0.0118641162030018
      | -0.0118927646086579
      | -0.0120000000000000
      | -0.0121897844459966
      | -0.0124393479427436
      | -0.0127192374681188
      | -0.0130000000000000
      | -0.0132593275201690
      | -0.0135034920260239
      | -0.0137459105188668
      | -0.0140000000000000
      | -0.0142729054733275
      | -0.0145466839531609
      | -0.0147971204564139
      | -0.0150000000000000
      | -0.0151334255865212
      | -0.0151847721613325
      | -0.0151437326554777
      | -0.0150000000000000
      | -0.0147402671805879
      | -0.0143392274015089
      | -0.0137685739216755
      | -0.0130000000000000
      | -0.0120148806911273
      | -0.0108333182326318
      | -0.00948509665782044
      | -0.00800000000000000
      | -0.00640333505490292
      | -0.00470249966796380
      | -0.00290041444704278
      | -0.00100000000000000
      | 0.000987595910738992
      | 0.00301831690448703
      | 0.00503987944599156
      | 0.00700000000000000
      | 0.00884357641194696
      | 0.0105042320500157
      | 0.0119127716630766
      | 0.0130000000000000
      | 0.0137162234414732
      | 0.0140897548954503
      | 0.0141684089017022
      | 0.0140000000000000
      | 0.0136196548221603
      | 0.0130117483681832
      | 0.0121479677301145
      | 0.0110000000000000
      | 0.00953953226988547
      | 0.00773825163181676
      | 0.00556784517783966
      | 0.00300000000000000]
  des_hip_torque [Nm] : Outport
  Disturbance velocity [deg/sec] : Outport  Port=2
  Out1 : Outport  Port=3
  wires:
  Sum1/1 -> Math Function1/1
  Math Function1/1 -> Gain4/1  "shifted gait percentage"
  Constant1/1 -> Math Function1/2
  ---> deg/sec/1 -> Disturbance velocity [deg/sec]/1
  Perturbation velocity (rad/sec)/1 -> ---> deg/sec/1
  Gain4/1 -> Perturbation velocity (rad/sec)/1
  Product1/1 -> ?  "unshifted_assistance torque"
  Embedded MATLAB Function1/1(Tout) -> Product1/1
  Gain2/1 -> winterAnkleFastSmooth3/1
  winterAnkleFastSmooth3/1 -> Embedded MATLAB Function1/1(T)
  Math Function/1 -> Gain1/1  "shifted gait percentage"
  Constant/1 -> Math Function/2
  Gain1/1 -> winterAnkleFastSmooth/1
  Product/1 -> des_hip_torque [Nm]/1
  Sum/1 -> Math Function/1
  gain_neg/1 -> Embedded MATLAB Function/3(gain_neg), Embedded MATLAB Function1/3(gain_neg)
  gain_pos/1 -> Embedded MATLAB Function/2(gain_pos), Embedded MATLAB Function1/2(gain_pos)
  Embedded MATLAB Function/1(Tout) -> Product/1
  winterAnkleFastSmooth/1 -> Embedded MATLAB Function/1(T)
  shift %/1 -> Sum1/2, Sum/2
  stride %/1 -> Sum/1, Gain2/1, Sum1/1
  Gain/1 -> Product/3, Product1/3
  assistance_level [%]/1 -> Gain/1
  body_weigth [Kg]/1 -> Product/2, Product1/2

== system MotorTorqueControlTest_working_5_8_2022_ADC_FILT_Mo/Subsystem1/HIGH LEVEL CONTROL (200 Hz)1/HIP_assistive_controller/stride % calculation ==
  step_trigger : Inport
  timer : Inport  Port=2
  step_freq_estimated : Inport  Port=3
  Product1 : Product  RndMeth=Zero
  Sum : Sum  Inputs=|-+
  take step start and period : Subsystem  TreatAsAtomicUnit=on
  to% : Gain  Gain=100  SampleTime=0.01
  step_start [s] : Outport
  freq_in_step [Hz] : Outport  Port=2
  stride % : Outport  Port=3
  wires:
  to%/1 -> stride %/1
  step_trigger/1 -> take step start and period/Trigger
  timer/1 -> take step start and period/1(time_counter), Sum/2
  take step start and period/1(time_count_stepon) -> step_start [s]/1, Sum/1
  step_freq_estimated/1 -> Product1/2, take step start and period/2(actual;_frequency)
  take step start and period/2(frequency for the step) -> freq_in_step [Hz]/1
  Sum/1 -> Product1/1
  Product1/1 -> to%/1

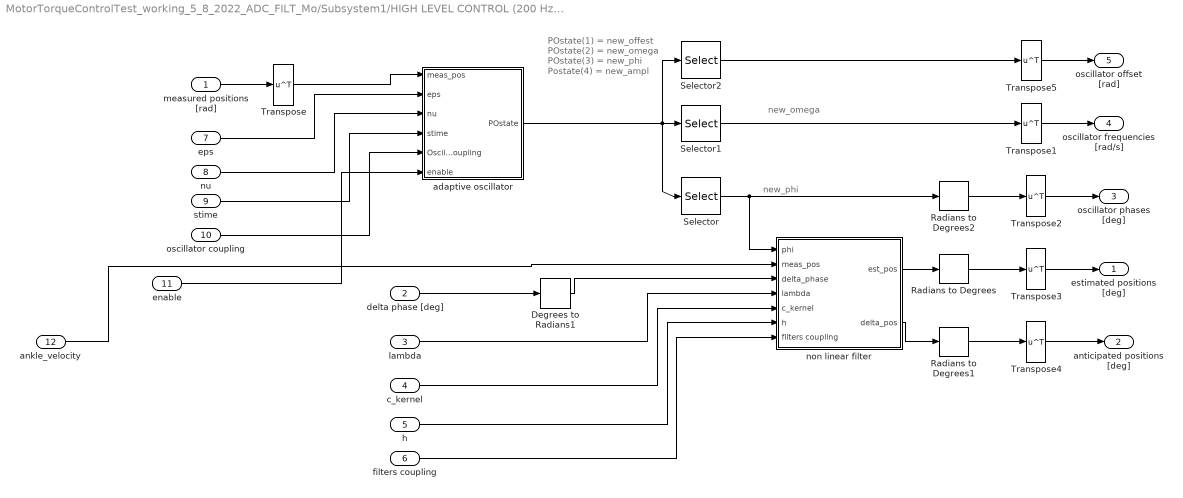
== system MotorTorqueControlTest_working_5_8_2022_ADC_FILT_Mo/Subsystem1/HIGH LEVEL CONTROL (200 Hz)1/non-linear AFO/non-linear adaptive oscillator ==
  note: new_phi
  note: new_omega
  note: POstate(1) = new_offest
      | POstate(2) = new_omega
      | POstate(3) = new_phi
      | Postate(4) = new_ampl
  measured positions [rad] : Inport
  delta phase [deg] : Inport  Port=2
  lambda : Inport  Port=3
  c_kernel : Inport  Port=4
  h : Inport  Port=5
  filters coupling : Inport  Port=6
  eps : Inport  Port=7
  nu : Inport  Port=8
  stime : Inport  Port=9
  oscillator coupling : Inport  Port=10
  enable : Inport  Port=11
  ankle_velocity : Inport  Port=12
  Degrees to Radians1 : simulink_extras/Transformations/Degrees to Radians
  Radians to Degrees : simulink_extras/Transformations/Radians to Degrees
  Radians to Degrees1 : simulink_extras/Transformations/Radians to Degrees
  Radians to Degrees2 : simulink_extras/Transformations/Radians to Degrees
  Selector : Selector  NumberOfDimensions=2  InputPortWidth=3  IndexOptions=Index vector (dialog),Index vector (dialog)  Indices=3,1:4  OutputSizes=1,1
  Selector1 : Selector  NumberOfDimensions=2  InputPortWidth=3  IndexOptions=Index vector (dialog),Index vector (dialog)  Indices=2,1:4  OutputSizes=1,1
  Selector2 : Selector  NumberOfDimensions=2  InputPortWidth=3  IndexOptions=Index vector (dialog),Index vector (dialog)  Indices=1,1:4  OutputSizes=1,1
  Transpose{,1..5} (6 alike) : Math  Operator=transpose
  adaptive oscillator : Subsystem
  non linear filter : Subsystem
  estimated positions [deg] : Outport
  anticipated positions [deg] : Outport  Port=2
  oscillator phases [deg] : Outport  Port=3
  oscillator frequencies [rad/s] : Outport  Port=4
  oscillator offset [rad] : Outport  Port=5
  wires:
  ankle_velocity/1 -> non linear filter/2(meas_pos)
  enable/1 -> adaptive oscillator/6(enable)
  Selector2/1 -> Transpose5/1
  Transpose5/1 -> oscillator offset [rad]/1
  oscillator coupling/1 -> adaptive oscillator/5(Oscillator coupling)
  stime/1 -> adaptive oscillator/4(stime)
  nu/1 -> adaptive oscillator/3(nu)
  eps/1 -> adaptive oscillator/2(eps)
  filters coupling/1 -> non linear filter/7(filters coupling)
  h/1 -> non linear filter/6(h)
  c_kernel/1 -> non linear filter/5(c_kernel)
  lambda/1 -> non linear filter/4(lambda)
  Degrees to Radians1/1 -> non linear filter/3(delta_phase)
  delta phase [deg]/1 -> Degrees to Radians1/1
  Transpose1/1 -> oscillator frequencies [rad/s]/1
  Transpose2/1 -> oscillator phases [deg]/1
  Transpose3/1 -> estimated positions [deg]/1
  Transpose4/1 -> anticipated positions [deg]/1
  Transpose/1 -> adaptive oscillator/1(meas_pos)
  Selector1/1 -> Transpose1/1
  Radians to Degrees2/1 -> Transpose2/1
  Radians to Degrees1/1 -> Transpose4/1
  Radians to Degrees/1 -> Transpose3/1
  measured positions [rad]/1 -> Transpose/1
  non linear filter/2(delta_pos) -> Radians to Degrees1/1
  non linear filter/1(est_pos) -> Radians to Degrees/1
  Selector/1 -> Radians to Degrees2/1, non linear filter/1(phi)
  adaptive oscillator/1(POstate) -> Selector2/1, Selector1/1, Selector/1

== system MotorTorqueControlTest_working_5_8_2022_ADC_FILT_Mo/Subsystem1/HIGH LEVEL CONTROL (200 Hz)1/HIP_assistive_controller/stride % calculation/take step start and period ==
  time_counter : Inport
  actual;_frequency : Inport  Port=2
  Trigger : TriggerPort  VariantControl=(inherit)
  time_count_stepon : Outport
  frequency for the step : Outport  Port=2
  wires:
  time_counter/1 -> time_count_stepon/1
  actual;_frequency/1 -> frequency for the step/1

== system MotorTorqueControlTest_working_5_8_2022_ADC_FILT_Mo/Subsystem1/HIGH LEVEL CONTROL (200 Hz)1/non-linear AFO/non-linear adaptive oscillator/adaptive oscillator ==
  note: eps = 6
      | nu = 0.25
      | stime = 0.001
  note: POstate(1) = new_offest
      | POstate(2) = new_omega
      | POstate(3) = new_phi
      | Postate(4) = new_ampl
  note: 0: no coupling
      | 1: hip coupled
      | 2: knee coupled
      | 3: hip and knee coupled
      | 4: right and left coupled
      | 5: all to all coupled
  meas_pos : Inport
  eps : Inport  Port=2
  nu : Inport  Port=3
  stime : Inport  Port=4
  Oscillator coupling : Inport  Port=5
  enable : Inport  Port=6
  Embedded MATLAB Function : MATLAB Function  TreatAsAtomicUnit=on  SystemSampleTime=0.002
  Mux : Mux  Inputs=3
  Unit Delay : UnitDelay  InitialCondition=repmat([0;pi/4;ones(6,1)*pi/2;ones(6,1)*0],1,4)  SampleTime=-1
  POstate : Outport
  wires:
  enable/1 -> Embedded MATLAB Function/5(enable)  "enable_AFO"
  stime/1 -> Mux/3
  nu/1 -> Mux/2
  eps/1 -> Mux/1
  Mux/1 -> Embedded MATLAB Function/2(parameters)
  Oscillator coupling/1 -> Embedded MATLAB Function/3(coupling)
  Unit Delay/1 -> Embedded MATLAB Function/4(POstate_in)
  Embedded MATLAB Function/1(POstate_out) -> Unit Delay/1, POstate/1  "PO_State"
  meas_pos/1 -> Embedded MATLAB Function/1(meas_pos)

== system MotorTorqueControlTest_working_5_8_2022_ADC_FILT_Mo/Subsystem1/HIGH LEVEL CONTROL (200 Hz)1/non-linear AFO/non-linear adaptive oscillator/non linear filter ==
  note: valori usati da renato:
      | lambda = 0.9999
      | c_kernel = (1:90)'/90* 2*pi
      | h = 1.6*90
      | filters coupling = 0
  note: 0: no coupling
      | 1: hip coupled
      | 2: knee coupled
      | 3: hip and knee coupled
  phi : Inport
  meas_pos : Inport  Port=2
  delta_phase : Inport  Port=3
  lambda : Inport  Port=4
  c_kernel : Inport  Port=5
  h : Inport  Port=6
  filters coupling : Inport  Port=7
  Embedded MATLAB Function : MATLAB Function  TreatAsAtomicUnit=on
  Unit Delay : UnitDelay  InitialCondition=zeros(90,4)  SampleTime=-1
  Unit Delay1 : UnitDelay  InitialCondition=ones(90,4)  SampleTime=-1
  est_pos : Outport
  delta_pos : Outport  Port=2
  wires:
  h/1 -> Embedded MATLAB Function/6(h)
  c_kernel/1 -> Embedded MATLAB Function/5(c_kernel)
  lambda/1 -> Embedded MATLAB Function/4(lambda)
  Embedded MATLAB Function/2(delta_pos) -> delta_pos/1
  Embedded MATLAB Function/1(est_pos) -> est_pos/1
  filters coupling/1 -> Embedded MATLAB Function/7(coupling)
  delta_phase/1 -> Embedded MATLAB Function/3(delta_phase)
  phi/1 -> Embedded MATLAB Function/2(phi)
  meas_pos/1 -> Embedded MATLAB Function/1(meas_pos)
  Unit Delay1/1 -> Embedded MATLAB Function/8(P_in)
  Embedded MATLAB Function/3(P_out) -> Unit Delay1/1
  Unit Delay/1 -> Embedded MATLAB Function/9(w_in)
  Embedded MATLAB Function/4(w_out) -> Unit Delay/1

== matlab function MotorTorqueControlTest_working_5_8_2022_ADC_FILT_Mo/MATLAB Function7 ==
  data: assistive_torque input; torque_cmd output; psum input; actual_angle input; assist_signal input; angle_threshold input; p_threshold input
function torque_cmd = torque_safety_cmd(assistive_torque, psum, actual_angle, assist_signal, angle_threshold, p_threshold)
%#codegen
% torque_safety_cmd
%   Simulink-friendly function:
%   - Uses persistent buffers for psum and angle
%   - Applies your pause_check and angle_safety_check logic
%   - Only outputs non-zero torque when conditions are satisfied

    %-----------------------------
    % Persistent state (kept between time steps)
    %-----------------------------
    persistent psum_buf angle_buf psum_idx angle_idx
    
    if isempty(psum_buf)
        % Initialize once at start of simulation
        PSUM_BUF_LEN   = 700;   % same idea as rem(i+1,1000)
        ANGLE_BUF_LEN  = 100;    % choose as you like
        
        psum_buf  = zeros(1, PSUM_BUF_LEN);
        angle_buf = zeros(1, ANGLE_BUF_LEN);
        psum_idx  = 0;
        angle_idx = 0;
    end

    %-----------------------------
    % 1) psum check (like pause_check)
    %-----------------------------
    psum_idx = mod(psum_idx, numel(psum_buf)) + 1;   % 1-based circular index
    psum_buf(psum_idx) = psum;

    if max(psum_buf) - min(psum_buf) < p_threshold
        psum_flag = 0;     % same logic as original function
    else
        psum_flag = 1;
    end

    %-----------------------------
    % 2) angle check (like angle_safety_check)
    %-----------------------------
    angle_idx = mod(angle_idx, numel(angle_buf)) + 1;
    angle_buf(angle_idx) = actual_angle;

    if max(angle_buf) - min(angle_buf) < angle_threshold
        angle_flag = 0;    % same logic as original function
    else
        angle_flag = 1;
    end

    %-----------------------------
    % 3) Combine with assistance signal → torque_cmd
    %-----------------------------
    % Here I assume "0" from the checks means SAFE/STABLE.
    % So we only pass assistance when:
    %   - assist_signal ~= 0
    %   - psum_flag  == 0
    %   - angle_flag == 0
    %
    % If in your existing model "1" means safe, just flip the
    % comparisons to (psum_flag == 1 && angle_flag == 1).
    if (assist_signal ~= 0) && (psum_flag == 0)
        torque_cmd = 0;   % let assistance through
    else
        torque_cmd = double(assist_signal) * assistive_torque;               % block torque
    end
end
